simulink model "SAR_ADC_new"  (R2021b)
settings: Solver=FixedStepAuto  StartTime=0.0  StopTime=100  FixedStep=1  RelTol=1e-3
libraries: simulink x1
settings Model: Creator=wilfred  LastModifiedBy=Pratham

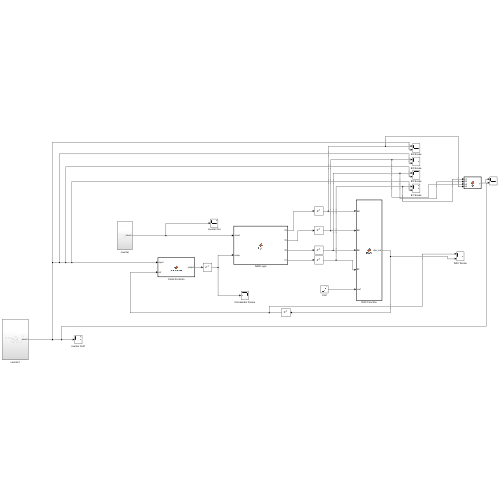
[thumbnail: Simulink's stored preview of the top-level diagram]
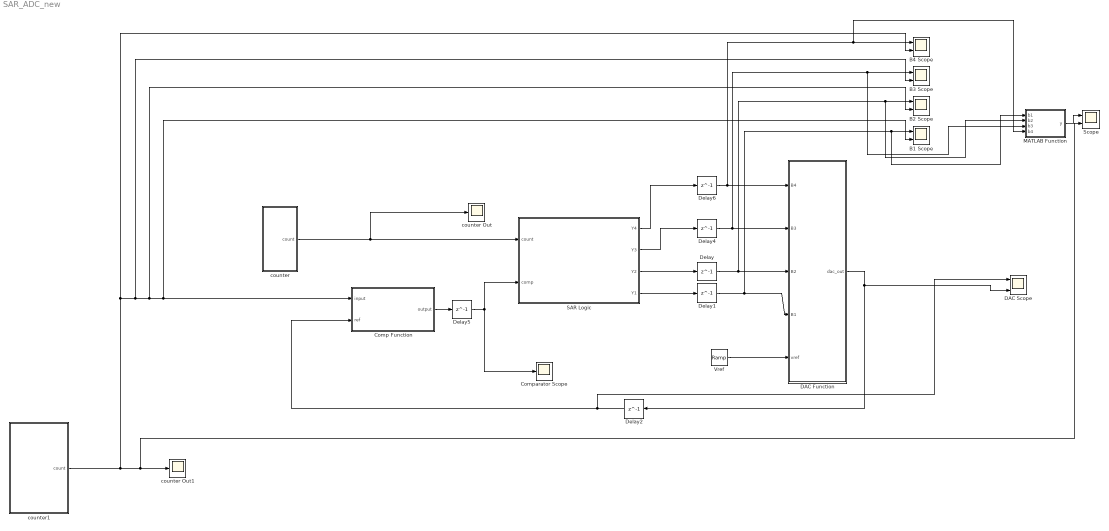
== system SAR_ADC_new ==
  B1 Scope : Scope  NumInputPorts=2
  B2 Scope : Scope  NumInputPorts=2
  B3 Scope : Scope  NumInputPorts=2
  B4 Scope : Scope  NumInputPorts=2
  Comp Function : MATLAB Function  TreatAsAtomicUnit=on
  Comparator Scope : Scope
  DAC Function : MATLAB Function  TreatAsAtomicUnit=on
  DAC Scope : Scope  NumInputPorts=2
  Delay{,1..2,4..6} (6 alike) : Delay  DelayLength=1  InitialCondition=0
  MATLAB Function : MATLAB Function  TreatAsAtomicUnit=on
  SAR Logic : MATLAB Function  TreatAsAtomicUnit=on
  Scope : Scope  NumInputPorts=2
  Vref : simulink/Sources/Ramp  slope=0  start=0  InitialOutput=1
  counter : Subsystem
  counter Out : Scope
  counter Out1 : Scope
  counter1 : Subsystem
  wires:
  DAC Function/1(dac_out) -> Delay2/1, DAC Scope/2
  Vref/1 -> DAC Function/5(vref)
  SAR Logic/4(Y1) -> Delay1/1
  Delay1/1 -> MATLAB Function/1(b1), B1 Scope/1, DAC Function/4(B1)
  SAR Logic/3(Y2) -> Delay/1
  Delay2/1 -> DAC Scope/1, Comp Function/2(ref)
  Comp Function/1(output) -> Delay5/1
  Delay5/1 -> Comparator Scope/1, SAR Logic/2(comp)
  counter/1(count) -> counter Out/1, SAR Logic/1(count)
  SAR Logic/2(Y3) -> Delay4/1
  SAR Logic/1(Y4) -> Delay6/1
  Delay6/1 -> MATLAB Function/4(b4), B4 Scope/1, DAC Function/1(B4)
  Delay4/1 -> MATLAB Function/3(b3), B3 Scope/1, DAC Function/2(B3)
  counter1/1(count) -> B4 Scope/2, Comp Function/1(input), B1 Scope/2, B2 Scope/2, B3 Scope/2, Scope/2, counter Out1/1
  Delay/1 -> MATLAB Function/2(b2), B2 Scope/1, DAC Function/3(B2)
  MATLAB Function/1(y) -> Scope/1

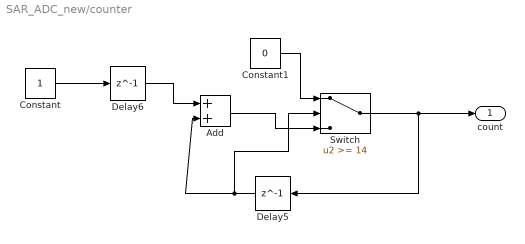
== system SAR_ADC_new/counter ==
  Add : Sum
  Constant : Constant
  Constant1 : Constant  Value=0
  Delay5 : Delay  DelayLength=1  InitialCondition=0
  Delay6 : Delay  DelayLength=1  InitialCondition=0
  Switch : Switch  Threshold=14
  count : Outport
  wires:
  Constant/1 -> Delay6/1
  Constant1/1 -> Switch/1
  Delay5/1 -> Switch/2, Add/2
  Add/1 -> Switch/3
  Switch/1 -> count/1, Delay5/1
  Delay6/1 -> Add/1

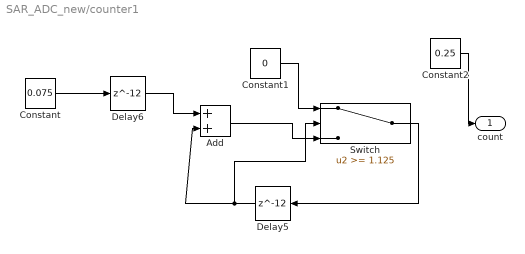
== system SAR_ADC_new/counter1 ==
  Add : Sum
  Constant : Constant  Value=0.075
  Constant1 : Constant  Value=0
  Constant2 : Constant  Value=0.25
  Delay5 : Delay  DelayLength=12  InitialCondition=0
  Delay6 : Delay  DelayLength=12  InitialCondition=0
  Switch : Switch  Threshold=1.125
  count : Outport
  wires:
  Constant/1 -> Delay6/1
  Constant1/1 -> Switch/1
  Delay5/1 -> Switch/2, Add/2
  Add/1 -> Switch/3
  Delay6/1 -> Add/1
  Switch/1 -> Delay5/1
  Constant2/1 -> count/1

== matlab function SAR_ADC_new/Comp Function ==
  data: input input; output output; ref input
function output = comparator(input, ref)


    if input >= ref
        output = 1;
    else 
        output = 0;
    end

== matlab function SAR_ADC_new/SAR Logic ==
  data: Y4 output; Y3 output; count input; Y2 output; comp input; Y1 output
function [Y4,Y3,Y2,Y1] = logic(count, comp)

persistent B3;
persistent B4;
persistent B2;
persistent B1;

if isempty(B4) && isempty(B3) && isempty(B2) && isempty(B1)
    B4 = 0b1;
    B3 = 0b0;
    B2 = 0b0;
    B1 = 0b0;
end

%%%%%%%%%%%%%%%%%%%%%%%%%%%%%
% if count == 3
%     if comp == 0b0
%         B2 = 0b0;
%         B1 = 0b1;
%     else
%         B2 = 0b1;
%         B1 = 0b1;
%     end
% end
% 
% if count == 6
%     if B2 == 0b0
%         if comp == 0b0
%             B1 = 0b0;
%         else
%             B1 = 0b1;
%         end
%     else
%         if comp == 0b0
%            B1 = 0b0;
%         else
%             B1 = 0b1;
%         end
%     end
% end
% 
% Y2 = B2;
% Y1 = B1;
% 
% if count == 6
%     B2 = 0b1;
%     B1 = 0b0;
% end

%%%%%%%%%%%%%%%%%%%%%%

if count == 3
    if comp == 0b0
        B4 = 0b0;
        B3 = 0b1;
        B2 = 0b0;
        B1 = 0b0;
    else
        B4 = 0b1;
        B3 = 0b1;
        B2 = 0b0;
        B1 = 0b0;
    end
end

if count == 6
    if B4 == 0b1
        if comp == 0b0
            B3 = 0b0;
            B2 = 0b1;
        else
            B3 = 0b1;
            B2 = 0b1;
        end
    else
        if comp == 0b0
            B3 = 0b0;
            B2 = 0b1;
        else
            B3 = 0b1;
            B2 = 0b1;
        end
    end
end

if count == 9
    if B3 == 0b1
        if comp == 0b0
            B2 = 0b0;
            B1 = 0b1;
        else
            B2 = 0b1;
            B1 = 0b1;
        end
    else
        if comp == 0b0
            B2 = 0b0;
            B1 = 0b1;
        else
            B2 = 0b1;
            B1 = 0b1;
        end
    end
end

if count == 12
    if B2 == 0b1
        if comp == 0b0
            B1 = 0b0;
        else
            B1 = 0b1;
        end
    else
        if comp == 0b0
            B1 = 0b0;
        else
            B1 = 0b1;
        end
    end
end

% if count == 12
%     if B2 == 0b1
%         if comp == 0b0
%             B1 = 0b0;
%         else
%             B1 = 0b1;
%         end
%     else
%         if comp == 0b0
%             B1 = 0b0;
%         else
%             B1 = 0b1;
%         end
%     end
% end

% if count == 12
%     if B2 == 0b1
%         if comp == 0b0
%             B1 = 0b0;
%         else
%             B1 = 0b1;
%         end
%     else
%         if comp == 0b0
%             B1 = 0b0;
%         else
%             B1 = 0b1;
%         end
%     end
% end

% if count == 12
%     if B2 == 0b1
%         if comp == 0b0
%             B1 = 0b0;
%         else
%             B1 = 0b1;
%         end
%     else
%         if comp == 0b0
%             B1 = 0b0;
%         else
%             B1 = 0b1;
%         end
%     end
% end

% if count == 12
%     if B2 == 0b1
%         if comp == 0b0
%             B1 = 0b0;
%         else
%             B1 = 0b1;
%         end
%     else
%         if comp == 0b0
%             B1 = 0b0;
%         else
%             B1 = 0b1;
%         end
%     end
% end

% if count == 12
%     if B2 == 0b1
%         if comp == 0b0
%             B1 = 0b0;
%         else
%             B1 = 0b1;
%         end
%     else
%         if comp == 0b0
%             B1 = 0b0;
%         else
%             B1 = 0b1;
%         end
%     end
% end

% if count == 12
%     if B2 == 0b1
%         if comp == 0b0
%             B1 = 0b0;
%         else
%             B1 = 0b1;
%         end
%     else
%         if comp == 0b0
%             B1 = 0b0;
%         else
%             B1 = 0b1;
%         end
%     end
% end

Y4 = B4;
Y3 = B3;
Y2 = B2;
Y1 = B1;

if count == 12
    B4 = 0b1;
    B3 = 0b0;
    B2 = 0b0;
    B1 = 0b0;
end

%%%%%%%%%%%%%%%%%%

== matlab function SAR_ADC_new/MATLAB Function ==
  data: b1 input; y output; b2 input; b3 input; b4 input
function y = fcn(b1,b2,b3,b4)
y = b1*(2^0) + b2*(2^1) + b3*(2^2) + b4*(2^3);

== matlab function SAR_ADC_new/DAC Function ==
  data: B4 input; B3 input; B2 input; dac_out output; B1 input; vref input
function dac_out = DAC(B4,B3,B2,B1,vref)

%binary representaion 0(b)MSB------LSB
%bin = dac_input;
%vec = bitget(bin, 1:1:8)


dac_out = vref * ((double(B4)/double(2^1)) + (double(B3)/double(2^2)) + (double(B2)/double(2^3)) + (double(B1)/double(2^4)));
